simulink model "pole_placement_model"  (R2022a)
settings: Solver=VariableStepAuto  StartTime=0.0  StopTime=25  MaxStep=1e-3  RelTol=1e-3
InitFcn:
  | clear
  | clc
  | %% dati
  | w0 = 5.278;
  | alfa1 = w0^2;
  | alfa3 = -1.402*w0^2;
  | alfa5 = 0.271*w0^2;
  | mu1 = 0.086;
  | mu3 = 0.1080;
  | %% matrici del sistema
  | A = [0 1; -alfa1 -2*mu1];
  | B = [0; 1];
  | C = [1 0];
  | D = [0; 0];
  | %% matrici sistema aumentato a causa dell'aggiunta dell'azione integrale
  | n = 2; % ordine del sistema
  | p = 1; % numero di uscite
  | Ag = [A zeros(n,p); -C 0];
  | Bg = [B; 0];
  | Ai=[A B; -C zeros(p,p)];
  | if rank(Ai)==n+p
  |    disp('Possiamo assegnare gli autovalori a ciclo chiuso, anche con l''aggiunta degli integratori')
  | end
  | %% assegnamento degli autovalori
  | p1 = -0.2;
  | p2 = -1.8;
  | p3 = -20;
  | p = [p1 p2 p3];
  | K = acker(Ag, Bg, p);
  | Kf = [K(1,1) K(1,2)];
  | Ki = K(1,3);
  | %% disturbi e variazioni parametriche
  | Ad = 0;
  | fd = 2;
  | alfa1_hat = 0.8*w0^2;
  | A_hat = [0 1; -alfa1_hat -2*mu1];
settings Model: Creator=user  LastModifiedBy=user

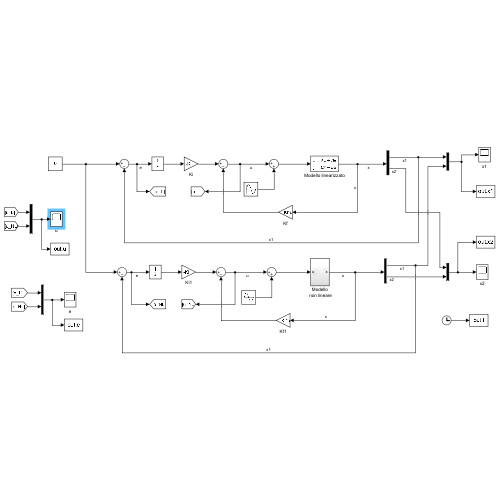
[thumbnail: Simulink's stored preview of the top-level diagram]
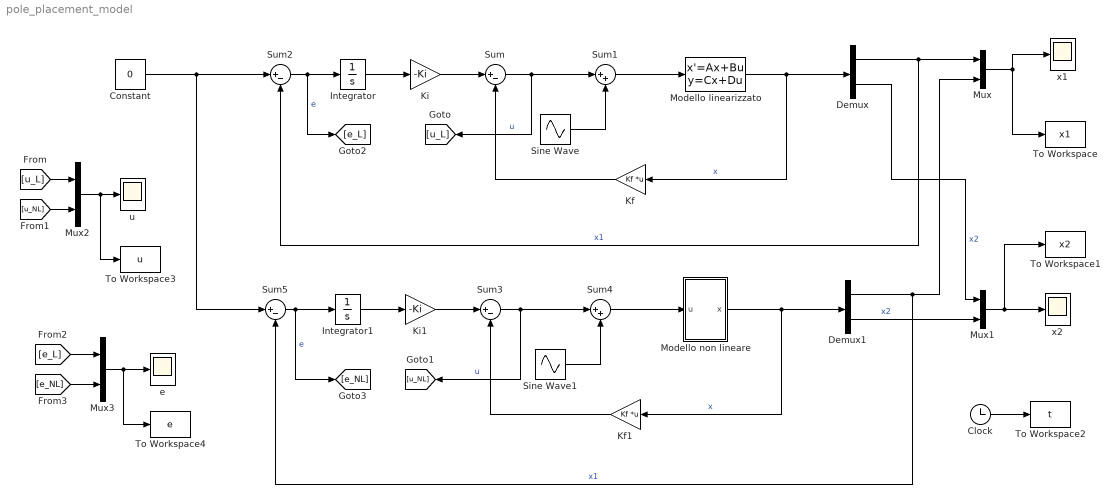
== system pole_placement_model ==
  Clock : Clock
  Constant : Constant  Value=0
  Demux : Demux  Outputs=2
  Demux1 : Demux  Outputs=2
  Integrator : Integrator
  Integrator1 : Integrator
  Kf : Gain  Gain=Kf  Multiplication=Matrix(K*u)
  Kf1 : Gain  Gain=Kf  Multiplication=Matrix(K*u)
  Ki : Gain  Gain=-Ki
  Ki1 : Gain  Gain=-Ki
  Modello non lineare : Subsystem
  Modello linearizzato : StateSpace  A=A  B=B  C=eye(2);  D=D  InitialCondition=[-1.2, -0.18]
  Mux{,1..3} (4 alike) : Mux  Inputs=2
  Sine Wave : Sin  Amplitude=Ad  Frequency=fd  SampleTime=0
  Sine Wave1 : Sin  Amplitude=Ad  Frequency=fd  SampleTime=0
  Sum{,2..3,5} (4 alike) : Sum  Inputs=|+-
  Sum1 : Sum  Inputs=|++
  Sum4 : Sum  Inputs=|++
  To Workspace : ToWorkspace  VariableName=x1  SampleTime=-1
      settings: Save2DSignal=2-D array (concatenate along first dimension)
  To Workspace1 : ToWorkspace  VariableName=x2  SampleTime=-1
      settings: Save2DSignal=2-D array (concatenate along first dimension)
  To Workspace2 : ToWorkspace  VariableName=t  SampleTime=-1
      settings: Save2DSignal=2-D array (concatenate along first dimension)
  To Workspace3 : ToWorkspace  VariableName=u  SampleTime=-1
      settings: Save2DSignal=2-D array (concatenate along first dimension)
  To Workspace4 : ToWorkspace  VariableName=e  SampleTime=-1
      settings: Save2DSignal=2-D array (concatenate along first dimension)
  e : Scope
  u : Scope
  x1 : Scope
  x2 : Scope
  wires:
  Constant/1 -> Sum5/1, Sum2/1
  Kf/1 -> Sum/2
  Modello linearizzato/1 -> Demux/1, Kf/1  "x"
  Sum/1 -> [u_L], Sum1/1  "u"
  Sum1/1 -> Modello linearizzato/1
  Sum2/1 -> [e_L], Integrator/1  "e"
  Demux/1 -> Sum2/2, Mux/1  "x1"
  Integrator/1 -> Ki/1
  Ki/1 -> Sum/1
  Sine Wave/1 -> Sum1/2
  Sine Wave1/1 -> Sum4/2
  Ki1/1 -> Sum3/1
  Integrator1/1 -> Ki1/1
  Modello non lineare/1(x) -> Demux1/1, Kf1/1  "x"
  Demux1/1 -> Sum5/2, Mux/2  "x1"
  Sum4/1 -> Modello non lineare/1(u)
  Sum5/1 -> [e_NL], Integrator1/1  "e"
  Kf1/1 -> Sum3/2
  Sum3/1 -> [u_NL], Sum4/1  "u"
  Mux/1 -> To Workspace/1, x1/1
  Mux1/1 -> To Workspace1/1, x2/1
  Demux1/2 -> Mux1/2  "x2"
  Demux/2 -> Mux1/1  "x2"
  Clock/1 -> To Workspace2/1
  [u_L] -> Mux2/1
  [u_NL] -> Mux2/2
  Mux2/1 -> To Workspace3/1, u/1
  [e_L] -> Mux3/1
  [e_NL] -> Mux3/2
  Mux3/1 -> To Workspace4/1, e/1

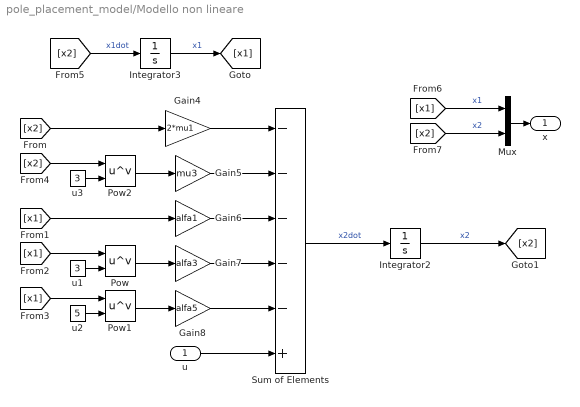
== system pole_placement_model/Modello non lineare ==
  u : Inport
  Gain4 : Gain  Gain=2*mu1
  Gain5 : Gain  Gain=mu3
  Gain6 : Gain  Gain=alfa1
  Gain7 : Gain  Gain=alfa3
  Gain8 : Gain  Gain=alfa5
  Integrator2 : Integrator  InitialCondition=-0.18
  Integrator3 : Integrator  InitialCondition=-1.2
  Mux : Mux  Inputs=2
  Pow : Math  Operator=pow  RndMeth=Zero
  Pow1 : Math  Operator=pow  RndMeth=Zero
  Pow2 : Math  Operator=pow  RndMeth=Zero
  Sum of Elements : Sum  Inputs=-----+
  u1 : Constant  Value=3
  u2 : Constant  Value=5
  u3 : Constant  Value=3
  x : Outport
  wires:
  Integrator3/1 -> [x1]  "x1"
  [x2] -> Gain4/1
  [x1] -> Pow/1
  Integrator2/1 -> [x2]  "x2"
  [x2] -> Pow2/1
  [x1] -> Gain6/1
  Mux/1 -> x/1
  [x1] -> Pow1/1
  Gain6/1 -> Sum of Elements/3
  [x1] -> Mux/1  "x1"
  u3/1 -> Pow2/2
  Pow2/1 -> Gain5/1
  u1/1 -> Pow/2
  [x2] -> Mux/2  "x2"
  Pow1/1 -> Gain8/1
  u2/1 -> Pow1/2
  Sum of Elements/1 -> Integrator2/1  "x2dot"
  [x2] -> Integrator3/1  "x1dot"
  Pow/1 -> Gain7/1
  Gain5/1 -> Sum of Elements/2
  Gain4/1 -> Sum of Elements/1
  Gain7/1 -> Sum of Elements/4
  u/1 -> Sum of Elements/6
  Gain8/1 -> Sum of Elements/5
